simulink model "M3_motor_load_gearbox_stiff"  (Simulink 10.2)
settings: Solver=FixedStepAuto  StartTime=0.0  StopTime=0.1  FixedStep=T_s*0.1  RelTol=1e-3
undefined symbols (not defined in the file): A_v, b_l, b_m, b_v, J_l, J_m, k, K_t, L, N_opt, omega_v, R, V_bar
settings Model: Creator=ioannis  LastModifiedBy=michelefocchi
settings DataIOCC: SaveFormat=Dataset  SignalLoggingSaveFormat=Dataset
settings OptimizationCC: LifeSpan=auto
settings DebuggingCC: UnderspecifiedInitializationDetection=Simplified  MergeDetectMultiDrivingBlocksExec=error  FcnCallInpInsideContextMsg=error  SFUnexpectedBacktrackingDiag=error  SFNoUnconditionalDefaultTransitionDiag=error  SFExecutionAtInitializationDiag=warning
settings HardwareCC: ProdBitPerPointer=64  ProdBitPerSizeT=64  ProdBitPerPtrDiffT=64  ProdLargestAtomicFloat=Float  ProdIntDivRoundTo=Zero  ProdEndianess=LittleEndian  ProdWordSize=64  ProdHWDeviceType=Intel->x86-64 (Windows64)
settings ModelReferenceCC: PropagateSignalLabelsOutOfModel=on
settings SFSimCC: SimUseLocalCustomCode=on
settings RTWCC: RTWUseLocalCustomCode=on
settings CodeAppCC: StateflowObjectComments=off
settings GRTTargetCC: TargetLangStandard=C99 (ISO)  CombineOutputUpdateFcns=on  GRTInterface=off
settings ConfigComp: CovMetricSettings=dwe  CovSaveCumulativeToWorkspaceVar=off  CovSaveSingleToWorkspaceVar=off  CovExternalEMLEnable=on

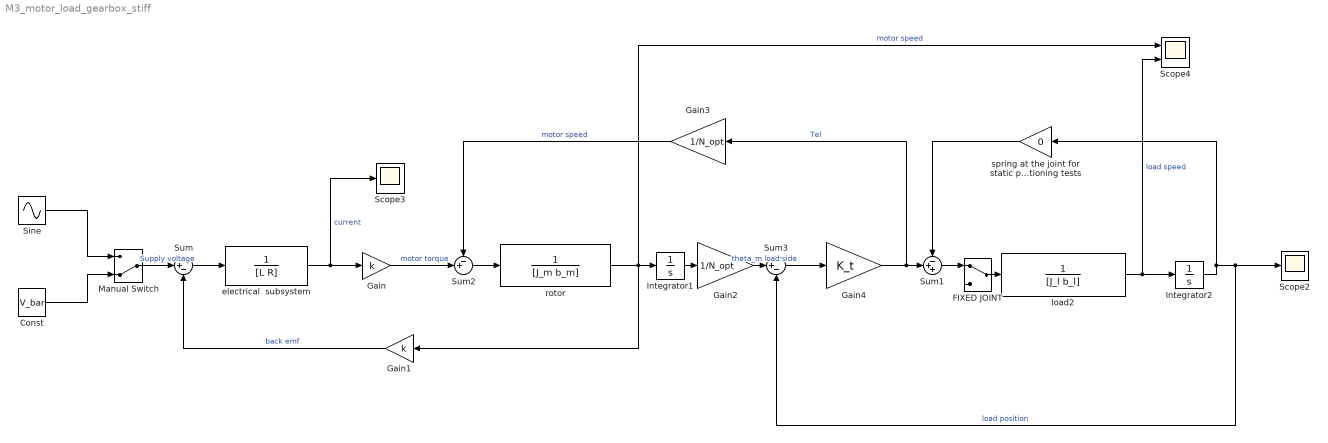
== system M3_motor_load_gearbox_stiff ==
  "Const " : Constant  Value=V_bar
  FIXED JOINT : ManualSwitch
  Gain : Gain  Gain=k
  Gain1 : Gain  Gain=k
  Gain2 : Gain  Gain=1/N_opt
  Gain3 : Gain  Gain=1/N_opt
  Gain4 : Gain  Gain=K_t
  Integrator1 : Integrator
  Integrator2 : Integrator
  Manual Switch : ManualSwitch  CurrentSetting=0
  Scope2 : Scope
  Scope3 : Scope
  Scope4 : Scope  NumInputPorts=2
  "Sine " : Sin  Amplitude=A_v  Bias=b_v  Frequency=omega_v  SampleTime=0
  Sum : Sum  Inputs=|+-
  Sum1 : Sum  Inputs=-++
  Sum2 : Sum  Inputs=-+|
  Sum3 : Sum  Inputs=|+-
  electrical  subsystem : TransferFcn  Denominator=[L R]
  load2 : TransferFcn  Denominator=[J_l b_l]
  rotor : TransferFcn  Denominator=[J_m b_m]
  spring at the joint for static positioning tests : Gain  Gain=0
  wires:
  Sum/1 -> electrical  subsystem/1
  Gain1/1 -> Sum/2  "back emf"
  electrical  subsystem/1 -> Gain/1, Scope3/1  "current"
  "Sine "/1 -> Manual Switch/1
  "Const "/1 -> Manual Switch/2
  Manual Switch/1 -> Sum/1  "Supply voltage"
  rotor/1 -> Gain1/1, Scope4/1, Integrator1/1  "motor speed"
  FIXED JOINT/1 -> load2/1
  Integrator1/1 -> Gain2/1
  Gain2/1 -> Sum3/1  "theta_m load side"
  Integrator2/1 -> Scope2/1, Sum3/2, spring at the joint for static positioning tests/1  "load position"
  load2/1 -> Scope4/2, Integrator2/1  "load speed"
  Sum1/1 -> FIXED JOINT/1
  Gain4/1 -> Gain3/1, Sum1/2  "Tel"
  Gain/1 -> Sum2/2  "motor torque"
  Sum2/1 -> rotor/1
  Gain3/1 -> Sum2/1  "motor speed"
  Sum3/1 -> Gain4/1
  spring at the joint for static positioning tests/1 -> Sum1/1
